simulink model "sys_ctrl_obs_luenberger_full_lineal_int_theta"  (Simulink 7.9)
settings: Solver=ode45  StartTime=0.0  StopTime=Tt  RelTol=1e-8
undefined symbols (not defined in the file): Ad, Bd, Cd, Dd, K, Knoise, L, max_alpha, max_dalpha, max_dtheta, max_theta, min_alpha, min_dalpha, min_dtheta, min_theta, Ts, x_0
settings Model: Creator=pdoren  LastModifiedBy=matias  CovModelRefEnable=off
settings SolverCC: ZeroCrossAlgorithm=Adaptive
settings DataIOCC: SaveFormat=StructureWithTime  SignalLoggingSaveFormat=Dataset
settings OptimizationCC: ExpressionDepthLimit=128
settings DebuggingCC: UnderspecifiedInitializationDetection=Simplified  MergeDetectMultiDrivingBlocksExec=error  SolverPrmCheckMsg=none  StateNameClashWarn=none
settings HardwareCC: ProdBitPerPointer=64  ProdLargestAtomicFloat=Float  ProdIntDivRoundTo=Zero  ProdEndianess=LittleEndian  ProdHWDeviceType=Specified
settings CodeAppCC: CustomSymbolStrType=$N$R$M_T
settings GRTTargetCC: CodeReplacementLibrary=C89/C90 (ANSI)  GeneratePreprocessorConditionals=Use local settings  CombineOutputUpdateFcns=off  GRTInterface=on

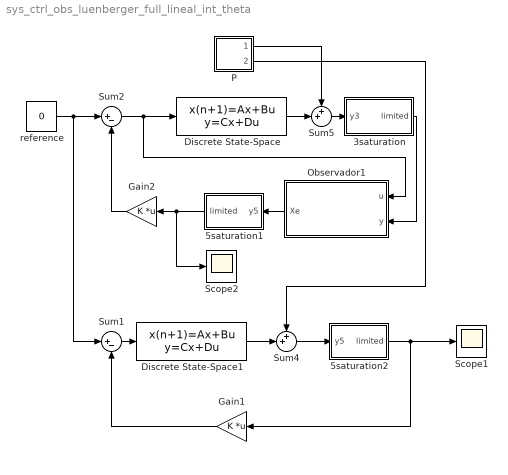
== system sys_ctrl_obs_luenberger_full_lineal_int_theta ==
  3saturation : Subsystem
  5saturation1 : Subsystem
  5saturation2 : Subsystem
  Discrete State-Space : DiscreteStateSpace  A=Ad  B=Bd  C=Cd  D=Dd  X0=x_0  SampleTime=Ts
  Discrete State-Space1 : DiscreteStateSpace  A=Ad  B=Bd  C=eye(5)  D=zeros(5,1)  X0=x_0  SampleTime=Ts
  Gain1 : Gain  Gain=K  Multiplication=Matrix(K*u)
  Gain2 : Gain  Gain=K  Multiplication=Matrix(K*u)
  Observador1 : Subsystem
  P : Subsystem
  Scope1 : Scope
      settings: YMin=-1.17714  YMax=3.02563  SaveName=states_lineal_d
  Scope2 : Scope
      settings: YMin=-1.17713  YMax=3.02585  SaveName=states_lineal_d_obs
  Sum1 : Sum  Inputs=|+-
  Sum2 : Sum  Inputs=|+-
  Sum4 : Sum  Inputs=++|
  Sum5 : Sum  Inputs=++|
  reference : Constant  Value=0
  wires:
  Sum2/1 -> Observador1/1(u), Discrete State-Space/1
  Gain2/1 -> Sum2/2
  Discrete State-Space/1 -> Sum5/2
  Sum5/1 -> 3saturation/1(y3)
  reference/1 -> Sum1/1, Sum2/1
  Sum1/1 -> Discrete State-Space1/1
  Gain1/1 -> Sum1/2
  Discrete State-Space1/1 -> Sum4/2
  Sum4/1 -> 5saturation2/1(y5)
  P/2(Noise5) -> Sum4/1
  P/1(Noise3) -> Sum5/1
  Observador1/1(Xe) -> 5saturation1/1(y5)
  3saturation/1(limited) -> Observador1/2(y)
  5saturation1/1(limited) -> Gain2/1, Scope2/1
  5saturation2/1(limited) -> Gain1/1, Scope1/1

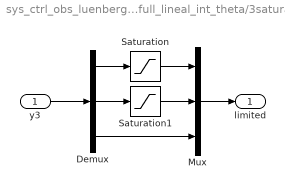
== system sys_ctrl_obs_luenberger_full_lineal_int_theta/3saturation ==
  y3 : Inport
  Demux : Demux  Outputs=3
  Mux : Mux  Inputs=3
  Saturation : Saturate  UpperLimit=max_theta  LowerLimit=min_theta
  Saturation1 : Saturate  UpperLimit=max_dalpha  LowerLimit=min_dalpha
  limited : Outport
  wires:
  y3/1 -> Demux/1
  Demux/1 -> Saturation/1
  Demux/2 -> Saturation1/1
  Saturation/1 -> Mux/1
  Saturation1/1 -> Mux/2
  Mux/1 -> limited/1
  Demux/3 -> Mux/3

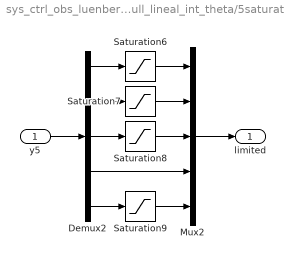
== system sys_ctrl_obs_luenberger_full_lineal_int_theta/5saturation1 ==
  y5 : Inport
  Demux2 : Demux  Outputs=5
  Mux2 : Mux  Inputs=5
  Saturation6 : Saturate  UpperLimit=max_alpha  LowerLimit=min_alpha
  Saturation7 : Saturate  UpperLimit=max_theta  LowerLimit=min_theta
  Saturation8 : Saturate  UpperLimit=max_dalpha  LowerLimit=min_dalpha
  Saturation9 : Saturate  UpperLimit=max_dtheta  LowerLimit=min_dtheta
  limited : Outport
  wires:
  Mux2/1 -> limited/1
  Saturation9/1 -> Mux2/5
  Demux2/5 -> Saturation9/1
  Demux2/4 -> Mux2/4
  Saturation8/1 -> Mux2/3
  Demux2/3 -> Saturation8/1
  Saturation7/1 -> Mux2/2
  Saturation6/1 -> Mux2/1
  Demux2/2 -> Saturation7/1
  Demux2/1 -> Saturation6/1
  y5/1 -> Demux2/1

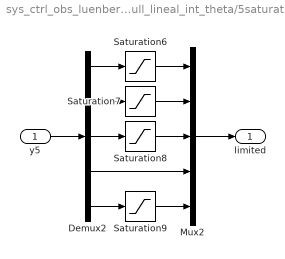
== system sys_ctrl_obs_luenberger_full_lineal_int_theta/5saturation2 ==
  y5 : Inport
  Demux2 : Demux  Outputs=5
  Mux2 : Mux  Inputs=5
  Saturation6 : Saturate  UpperLimit=max_alpha  LowerLimit=min_alpha
  Saturation7 : Saturate  UpperLimit=max_theta  LowerLimit=min_theta
  Saturation8 : Saturate  UpperLimit=max_dalpha  LowerLimit=min_dalpha
  Saturation9 : Saturate  UpperLimit=max_dtheta  LowerLimit=min_dtheta
  limited : Outport
  wires:
  Mux2/1 -> limited/1
  Saturation9/1 -> Mux2/5
  Demux2/5 -> Saturation9/1
  Demux2/4 -> Mux2/4
  Saturation8/1 -> Mux2/3
  Demux2/3 -> Saturation8/1
  Saturation7/1 -> Mux2/2
  Saturation6/1 -> Mux2/1
  Demux2/2 -> Saturation7/1
  Demux2/1 -> Saturation6/1
  y5/1 -> Demux2/1

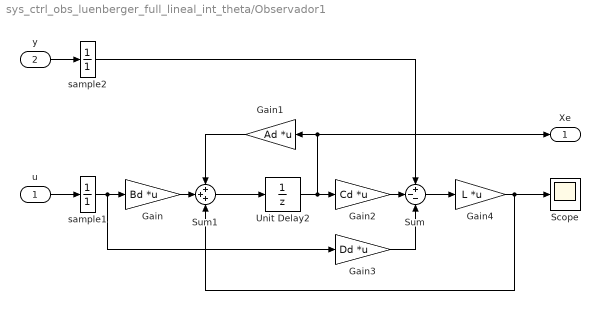
== system sys_ctrl_obs_luenberger_full_lineal_int_theta/Observador1 ==
  u : Inport
  y : Inport  Port=2
  Gain : Gain  Gain=Bd  Multiplication=Matrix(K*u)
  Gain1 : Gain  Gain=Ad  Multiplication=Matrix(K*u)
  Gain2 : Gain  Gain=Cd  Multiplication=Matrix(K*u)
  Gain3 : Gain  Gain=Dd  Multiplication=Matrix(K*u)
  Gain4 : Gain  Gain=L  Multiplication=Matrix(K*u)
  Scope : Scope
      settings: YMin=-30.481  YMax=47.09183
  Sum : Sum  Inputs=+--
  Sum1 : Sum  Inputs=+++
  Unit Delay2 : UnitDelay  SampleTime=Ts
  sample1 : DiscreteTransferFcn  Denominator=[1]  SampleTime=Ts
  sample2 : DiscreteTransferFcn  Denominator=[1]  SampleTime=Ts
  Xe : Outport
  wires:
  Unit Delay2/1 -> Gain2/1, Xe/1, Gain1/1
  u/1 -> sample1/1
  sample1/1 -> Gain/1, Gain3/1
  Sum/1 -> Gain4/1
  y/1 -> sample2/1
  sample2/1 -> Sum/1
  Gain3/1 -> Sum/3
  Gain2/1 -> Sum/2
  Gain/1 -> Sum1/2
  Gain4/1 -> Sum1/3, Scope/1
  Gain1/1 -> Sum1/1
  Sum1/1 -> Unit Delay2/1

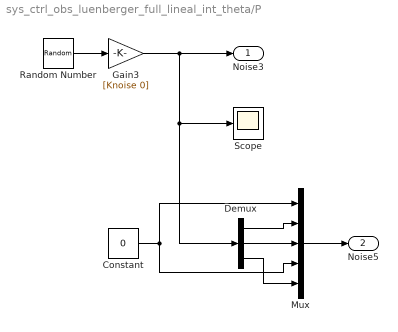
== system sys_ctrl_obs_luenberger_full_lineal_int_theta/P ==
  Constant : Constant  Value=0
  Demux : Demux  Outputs=3
  Gain3 : Gain  Gain=[Knoise 0]
  Mux : Mux  Inputs=5
  Random Number : RandomNumber  SampleTime=Ts
  Scope : Scope
      settings: YMin=-1.00000  YMax=1.00000
  Noise3 : Outport
  Noise5 : Outport  Port=2
  wires:
  Random Number/1 -> Gain3/1
  Gain3/1 -> Noise3/1, Demux/1, Scope/1
  Mux/1 -> Noise5/1
  Demux/1 -> Mux/2
  Demux/2 -> Mux/3
  Constant/1 -> Mux/4, Mux/1
  Demux/3 -> Mux/5
